simulink model "stewart_active_damping"  (R2019b)
settings: Solver=ode23s  StartTime=0.0  StopTime=10.0  FixedStep=1e-3  RelTol=1e-3  AbsTol=1e-3
libraries: nesl_utility x7, sm_lib x4
settings Model: Creator=thomas  LastModifiedBy=thomas
settings SolverCC: AutoScaleAbsTol=off
settings DebuggingCC: SymbolicDimsDataTypeCodeGenerationDiagnostic=none
settings SFSimCC: CustomCodeUndefinedFunction=UseInterfaceOnly
settings SimscapeCC: SimscapeLogType=all  SimscapeLogSimulationStatistics=on  SimscapeLogDataHistory=10000

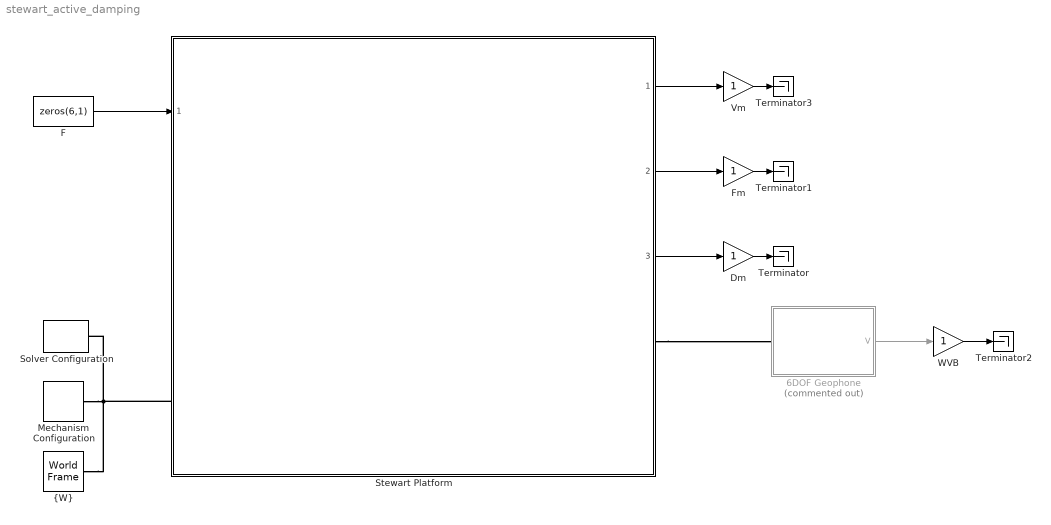
== system stewart_active_damping ==
  6DOF Geophone : Subsystem  Commented=on
  Dm : Gain
  F : Constant  Value=zeros(6,1)
  Fm : Gain
  Mechanism Configuration : sm_lib/Utilities/Mechanism Configuration  UniformGravity=None  GravityVector=[0 0 0]  GravityUnits=m/s^2  LinearizationDelta=1e-6
  Solver Configuration : nesl_utility/Solver Configuration  PhysicalDomain=network_engine_domain  SubClassName=solver  LeftPortType=input  RightPortType=generic  Tones=[]  Harmonics=[]  SimulateNoise=off  Profile=off  UseLocalSampling=off  EnableSwitchedLinearOptims=on  FrequencyDomain=off  UseCCode=off  RelTol=0.001  AbsTol=1e-06  MinStep=1e-09  ToWorkspace=off  RevertToSquareIcSolve=off  NumHomotopyIterations=100  PhasorMode=off  PhasorModeNumHarmonics=1  DoDC=off  ResidualTolerance=1e-09  UseLocalSolver=off  LocalSolverChoice=NE_BACKWARD_EULER_ADVANCER  LocalSolverSampleTime=0.001  DoFixedCost=off  MaxNonlinIter=3  MaxModeIter=2  LinearAlgebra=auto  EquationFormulation=NE_TIME_EF  DelaysMemoryBudget=1024  AutomaticFiltering=on  FilteringTimeConstant=0.001  PartitionStorageMethod=AS_NEEDED  PartitionMemoryBudget=1024  PartitionMethod=ROBUST
  Stewart Platform : Subsystem  ReferencedSubsystem=Stewart_Platform
  Terminator{,1..3} (4 alike) : Terminator
  Vm : Gain
  WVB : Gain
  "{W}" : sm_lib/Frames and Transforms/World Frame
  wires:
  WVB/1 -> Terminator2/1
  Fm/1 -> Terminator1/1
  Dm/1 -> Terminator/1
  6DOF Geophone/1(V) -> WVB/1
  Vm/1 -> Terminator3/1
  F/1 -> Stewart Platform/1
  Stewart Platform/1 -> Vm/1
  Stewart Platform/2 -> Fm/1
  Stewart Platform/3 -> Dm/1
  connections:
  "{W}"/RConn1 -- Stewart Platform/LConn2 -- Solver Configuration/RConn1 -- Mechanism Configuration/RConn1
  Stewart Platform/RConn1 -- 6DOF Geophone/LConn1

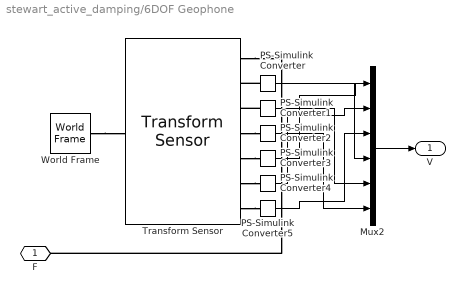
== system stewart_active_damping/6DOF Geophone ==
  Mux2 : Mux  Inputs=6
  PS-Simulink Converter{,1..5} (6 alike) : nesl_utility/PS-Simulink Converter  PhysicalDomain=network_engine_domain  SubClassName=ps_output  LeftPortType=input  RightPortType=output  PseudoPeriodic=off  Frequencies=[]  Unit=inherit  AffineConversion=off
  Transform Sensor : sm_lib/Frames and Transforms/Transform Sensor  MeasurementFrame=World  SenseAngle=off  SenseAxis=off  SenseAngle1=off  SenseAngle2=off  SenseAngle3=off  SenseQ=off  SenseR=off  SenseOmegaX=on  SenseOmegaY=on  SenseOmegaZ=on  SenseOmega1=off  SenseOmega2=off  SenseOmega3=off  SenseQDot=off  SenseRDot=off  SenseAlphaX=off  SenseAlphaY=off  SenseAlphaZ=off  SenseAlpha1=off  SenseAlpha2=off  SenseAlpha3=off  SenseQDDot=off  SenseRDDot=off  SenseX=off  SenseY=off  SenseZ=off  SenseRad=off  SenseAzim=off  SenseDist=off  SenseInc=off  SenseXDot=on  SenseYDot=on  SenseZDot=on  SenseRadDot=off  SenseAzimDot=off  SenseDistDot=off  SenseIncDot=off  SenseXDDot=off  SenseYDDot=off  SenseZDDot=off  SenseRadDDot=off  SenseAzimDDot=off  SenseDistDDot=off  SenseIncDDot=off
  World Frame : sm_lib/Frames and Transforms/World Frame
  F : PMIOPort  Side=Left
  V : Outport
  wires:
  PS-Simulink Converter2/1 -> Mux2/6
  PS-Simulink Converter1/1 -> Mux2/5
  PS-Simulink Converter/1 -> Mux2/4
  PS-Simulink Converter3/1 -> Mux2/1
  Mux2/1 -> V/1
  PS-Simulink Converter4/1 -> Mux2/2
  PS-Simulink Converter5/1 -> Mux2/3
  connections:
  Transform Sensor/RConn5 -- PS-Simulink Converter3/LConn1
  Transform Sensor/RConn4 -- PS-Simulink Converter2/LConn1
  PS-Simulink Converter1/LConn1 -- Transform Sensor/RConn3
  Transform Sensor/RConn6 -- PS-Simulink Converter4/LConn1
  Transform Sensor/RConn7 -- PS-Simulink Converter5/LConn1
  Transform Sensor/RConn1 -- F/RConn1
  PS-Simulink Converter/LConn1 -- Transform Sensor/RConn2
  World Frame/RConn1 -- Transform Sensor/LConn1
